simulink model "SIM_PEM"  (R2020b)
settings: Solver=ode23tb  StartTime=0.0  StopTime=3600  RelTol=1e-4  AbsTol=1e-3  EnableMultiTasking=on
undefined symbols (not defined in the file or in its folder): DiscIntNeverNeededParam, FC, FuelCellLoadFcn, gcbh, sps_rtmsupport
libraries: powerlib x16, spsFuelCellModel x1, simulink x1
settings Model: Creator=MathWorks  LastModifiedBy=janluca
settings SolverCC: AutoScaleAbsTol=off
settings DataIOCC: LimitDataPoints=on  SaveFormat=Array  SignalLoggingSaveFormat=ModelDataLogs  ReturnWorkspaceOutputs=off
settings OptimizationCC: ExpressionDepthLimit=2147483647  InitFltsAndDblsToZero=on  EfficientMapNaN2IntZero=off  LifeSpan=inf
settings DebuggingCC: SaveWithParameterizedLinksMsg=none  UnderspecifiedInitializationDetection=Classic  MergeDetectMultiDrivingBlocksExec=none  FcnCallInpInsideContextMsg=warning  AllowSymbolicDim=off  StateNameClashWarn=warning  SFUnexpectedBacktrackingDiag=warning  SFNoUnconditionalDefaultTransitionDiag=warning  SFExecutionAtInitializationDiag=none  ArithmeticOperatorsInVariantConditions=warning
settings HardwareCC: ProdBitPerPointer=32  ProdBitPerSizeT=32  ProdBitPerPtrDiffT=32  ProdLargestAtomicFloat=None  ProdIntDivRoundTo=Undefined  ProdEndianess=Unspecified  ProdWordSize=32  ProdHWDeviceType=32-bit Generic
settings ModelReferenceCC: PropagateSignalLabelsOutOfModel=off
settings SFSimCC: SimUseLocalCustomCode=off  CustomCodeUndefinedFunction=UseInterfaceOnly
settings RTWCC: RTWUseLocalCustomCode=off
settings CodeAppCC: StateflowObjectComments=on
settings GRTTargetCC: TargetFcnLib=ansi_tfl_tmw.mat  TargetLangStandard=C89/C90 (ANSI)  CombineOutputUpdateFcns=off  GRTInterface=on
settings ConfigComp: CovMetricSettings=dw  CovSaveCumulativeToWorkspaceVar=on  CovSaveSingleToWorkspaceVar=on  CovExternalEMLEnable=off  CovSFcnEnable=off
settings SimscapeCC: SimscapeNormalizeSystem=off

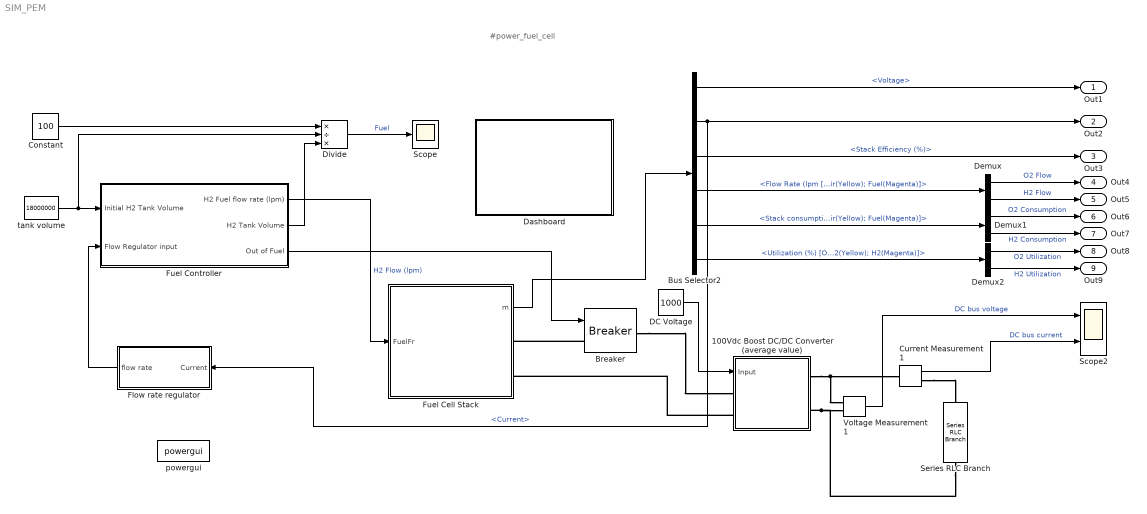
== system SIM_PEM ==
  note: #power_fuel_cell
  100Vdc Boost DC/DC Converter (average value) : Subsystem
  Breaker : powerlib/Elements/Breaker  InitialState=1  SwitchingTimes="[1/60  5/60]"  External=on  BreakerResistance=0.01  SnubberResistance=1e6  SnubberCapacitance=inf  Measurements=None  MoreParameters=on  NoBreakLoop=off
  Bus Selector2 : BusSelector  OutputSignals=Voltage,Current,Stack Efficiency (%),Flow Rate (lpm [Air(Yellow); Fuel(Magenta)],Stack consumption (Standard lpm) [Air(Yellow); Fuel(Magenta)],Utilization (%) [O2(Yellow); H2(Magenta)]
  Constant : Constant  Value=100
  Current Measurement1 : powerlib/Measurements/Current Measurement  PhasorSimulation=off  OutputType=Complex  PSBequivalent=0
  DC Voltage : Constant  Value=1000
  Dashboard : Subsystem
  Demux : Demux  Outputs=2
  Demux1 : Demux  Outputs=2
  Demux2 : Demux  Outputs=2
  Divide : Product  Inputs=*/*
  Flow rate regulator : Subsystem  mask{Nc=96, Uf_H2=99.18, T=65, Pf=1, x=99.95}
      mask prompts: Nc "Number of cells"; Uf_H2 "Nominal Hydrogen utilization (%)"; T "Operating temperature (Celsius)"; Pf "Fuel pressure (bar)"; x "H2 composition (%)"
  Fuel Cell Stack : Subsystem  AncestorBlock=electricdrivelib/Extra Sources/Fuel Cell Stack  DialogController=POWERSYS.PowerSysDialog  LoadFcn=sps_rtmsupport('LoadFcn',gcbh);FuelCellLoadFcn(gcb)  StartFcn=sps_rtmsupport('StartFcn',gcbh);  StopFcn=sps_rtmsupport('StopFcn',gcbh);  mask(Fuel Cell Stack){PresetModel=No (User-Defined), FcType=Proton Exchange Membrane (PEM), Detailed=Detailed, Eoc=[93.2,88], NomVI=[160,65.5], EndVI=[230,58.6], Nc=96, n=54, TOp=65, AirFr=510, SuppPress=[1.26,1], Comp=[99.95,21,1], SignX=off, SignY=off, FlowRateH2=on, FlowRateAir=off, SystemTemp=off, SystemPH2=off, SystemPAir=off, FCDyn=off, FC_tau=0, Peak_O2=80, V_Under=10}
      mask prompts: PresetModel "Preset model:"; FcType "Fuel Cell type:"; Detailed "Model detail Level:"; Eoc "Voltage at 0A and 1A [V_0(V), V_1(V)]"; NomVI "Nominal operating point [Inom(A), Vnom(V)]"; EndVI "Maximum operating point [Iend(A), Vend(V)]"; Nc "Number of cells"; n "Nominal stack efficiency (%)"; TOp "Operating temperature (Celsius)"; AirFr "Nominal Air flow rate (lpm)"; SuppPress "Nominal supply pressure [Fuel (bar), Air (bar)]"; Comp "Nominal composition (%) [H2 O2 H2O(Air)]"; SignX "Fuel  composition [x_H2(%)]"; SignY "Oxidant composition [y_O2(%)]"; FlowRateH2 "Fuel flow rate [FuelFr(lpm)]"; FlowRateAir "Air flow rate [AirFr(lpm)]"; SystemTemp "System Temperature [T(Kelvin)]"; SystemPH2 "Fuel supply pressure [Pfuel(bar)]"; SystemPAir "Air supply pressure [PAir(bar)]"; FCDyn "Specify Fuel Cell Dynamics?"; FC_tau "Fuel Cell response time (sec)"; Peak_O2 "Peak O2 utilization (%)"; V_Under "Voltage undershoot (V) @ peak O2 utilization"
      mask help:
      | Implements a generic hydrogen fuel cell model which allows the simulation for the following types of cells:
      | - Proton Exchange Membrane Fuel Cell (PEMFC)
      | - Solid Oxide Fuel Cell (SOFC)
      | - Alkaline Fuel Cell (AFC)
      mask init:
      | block = gcb;
      | %% DO NOT CHANGE THIS ORDER
      | FuelCellCback(block,'Inputs')
      | [FC, WantBlockChoice, Ts] = FuelCellInit(block,Eoc,NomVI,EndVI,Nc,n,TOp,AirFr,SuppPress,Comp,FlowRateH2,FlowRateAir);
      | powericon('SetInternalModels','set',block,WantBlockChoice);
      settings: CopyFcn=sps_rtmsupport('CopyFcn',gcbh);  DeleteFcn=sps_rtmsupport('DeleteFcn',gcbh);  UndoDeleteFcn=sps_rtmsupport('UndoDeleteFcn',gcbh);  ModelCloseFcn=sps_rtmsupport('ModelCloseFcn',gcbh);  PreSaveFcn=sps_rtmsupport('PreSaveFcn',gcbh);  PostSaveFcn=sps_rtmsupport('PostSaveFcn',gcbh);  NameChangeFcn=sps_rtmsupport('NameChangeFcn',gcbh);  PreCopyFcn=sps_rtmsupport('PreCopyFcn',gcbh);  OpenFcn=sps_rtmsupport('OpenFcn',gcbh, [1 2 3 13 14 15 16 17 18 19 20]);  CloseFcn=sps_rtmsupport('CloseFcn',gcbh);  PreDeleteFcn=sps_rtmsupport('PreDeleteFcn',gcbh);
      mask Help: helpview(psbhelp)
      mask TypeOptions PresetModel: No (User-Defined) | PEMFC - 1.26 kW - 24 Vdc | PEMFC - 6 kW - 45 Vdc | PEMFC - 50 kW - 625 Vdc | AFC - 2.4 kW - 48 Vdc | SOFC - 3 kW - 100 Vdc | SOFC - 25 kW - 630 Vdc
      mask Callback PresetModel: FuelCellCback(gcb,'Preset')
      mask TypeOptions Detailed: Simplified | Detailed
      mask Callback Detailed: FuelCellCback(gcb,'Visibilities')
      mask Callback FlowRateAir: FuelCellCback(gcb,'Visibilities')
      mask Callback FCDyn: FuelCellCback(gcb,'Visibilities')
      mask DialogControl ParameterTabVar0 Prompt: Parameters
      mask DialogControl plot_graph Prompt: Plot V_I characteristic
      mask DialogControl plot_graph Callback: FuelCellCback(gcb,'PlotGraph');
      mask DialogControl ViewParam Prompt: View Cell parameters
      mask DialogControl ViewParam Callback: FuelCellCback(gcb,'ViewParam');
      mask DialogControl ParameterTabVar01 Prompt: Signal variation
      mask DialogControl ParameterTabVar012 Prompt: Fuel Cell Dynamics
      mask Display: image(imread('power_fuelcell.png'));
  Fuel Controller : Subsystem
  Scope : Scope
  Scope2 : Scope  NumInputPorts=2
  Series RLC Branch : powerlib/Elements/Series RLC Branch  LConnTagsString=__new0  RConnTagsString=__new0  BranchType=R  Resistance=150  Inductance=100*100/6000  SetiL0=off  InitialCurrent=0  Capacitance=1e-6  Setx0=off  InitialVoltage=0  Measurements=None
  Voltage Measurement1 : powerlib/Measurements/Voltage Measurement  PhasorSimulation=off  OutputType=Complex  PSBequivalent=0
  powergui : powerlib/powergui  SimulationMode=Continuous  SampleTime=1e-5  frequency=50  Iterations=50  frequencyindice=0  Pbase=100e6  ErrMax=1e-4  UnitsV=kV  UnitsW=MW  buscounter=0  FunctionMessages=off  echomessages=off  EnableUseOfTLC=off  CurrentSourceSwitches=off  DisableSnubberDevices=off  DisableRonSwitches=off  DisableVfSwitches=off  DisplayEquations=off  AutomaticDiscreteSolvers=off  SolverType=Tustin  Interpol=off  ExternalGateDelay=off  methode=off  Ts=0  x0status=blocks  SPID=off  SwTol=0  HookPort=off  NonlinearTolerance=1e-4  nMaxIteration=100  ContinueOnMaxIteration=off  RestoreLinks=warning  ResistiveCurrentMeasurement=off  Frange=[0:2:500]  Ylog=off  Xlog=on  ShowGrid=off  save=off  variable=ZData  structure=0  ZoomFFT=on  StartTime=0.0  cycles=1  DisplayStyle=1  fundamental=60  FreqAxis=off  MaxFrequency=1000  frequencyindicesteady=1  RmsSteady=1  display=off
  tank volume : Constant  Value=18000000
  Out1 : Outport  SignalName=Stack Voltage
  Out2 : Outport  Port=2  SignalName=Stack Current
  Out3 : Outport  Port=3  SignalName=Stack Efficiency
  Out4 : Outport  Port=4  SignalName=O2 Flow
  Out5 : Outport  Port=5  SignalName=H2 Flow
  Out6 : Outport  Port=6  SignalName=O2 Consumption
  Out7 : Outport  Port=7  SignalName=H2 Consumption
  Out8 : Outport  Port=8  SignalName=O2 Utilization
  Out9 : Outport  Port=9  SignalName=H2 Utilization
  wires:
  Fuel Cell Stack/1(m) -> Bus Selector2/1
  Current Measurement1/1 -> Scope2/2  "DC bus current"
  Fuel Controller/1(H2 Fuel flow rate (lpm)) -> Fuel Cell Stack/1(FuelFr)  "H2 Flow (lpm)"
  tank volume/1 -> Divide/2, Fuel Controller/1(Initial H2 Tank Volume)
  Flow rate regulator/1(flow rate) -> Fuel Controller/2(Flow Regulator input)
  Fuel Controller/3(Out of Fuel) -> Breaker/1
  Bus Selector2/4 -> Demux/1  "<Flow Rate (lpm [Air(Yellow); Fuel(Magenta)]>"
  Bus Selector2/5 -> Demux1/1  "<Stack consumption (Standard lpm) [Air(Yellow); Fuel(Magenta)]>"
  Bus Selector2/6 -> Demux2/1  "<Utilization (%) [O2(Yellow); H2(Magenta)]>"
  Bus Selector2/1 -> Out1/1  "<Voltage>"
  Bus Selector2/2 -> Out2/1, Flow rate regulator/1(Current)  "<Current>"
  Bus Selector2/3 -> Out3/1  "<Stack Efficiency (%)>"
  Demux/1 -> Out4/1  "O2 Flow"
  Demux/2 -> Out5/1  "H2 Flow"
  Demux1/1 -> Out6/1  "O2 Consumption"
  Demux1/2 -> Out7/1  "H2 Consumption"
  Demux2/1 -> Out8/1  "O2 Utilization"
  Demux2/2 -> Out9/1  "H2 Utilization"
  Divide/1 -> Scope/1  "Fuel"
  Fuel Controller/2(H2 Tank Volume) -> Divide/3
  Constant/1 -> Divide/1
  Voltage Measurement1/1 -> Scope2/1  "DC bus voltage"
  DC Voltage/1 -> 100Vdc Boost DC/DC Converter (average value)/1(Input)
  connections:
  100Vdc Boost DC/DC Converter (average value)/RConn2 -- Series RLC Branch/RConn1 -- Voltage Measurement1/LConn2
  Current Measurement1/RConn1 -- Series RLC Branch/LConn1
  100Vdc Boost DC/DC Converter (average value)/LConn2 -- Fuel Cell Stack/RConn2
  Breaker/RConn1 -- 100Vdc Boost DC/DC Converter (average value)/LConn1
  100Vdc Boost DC/DC Converter (average value)/RConn1 -- Current Measurement1/LConn1 -- Voltage Measurement1/LConn1
  Breaker/LConn1 -- Fuel Cell Stack/RConn1

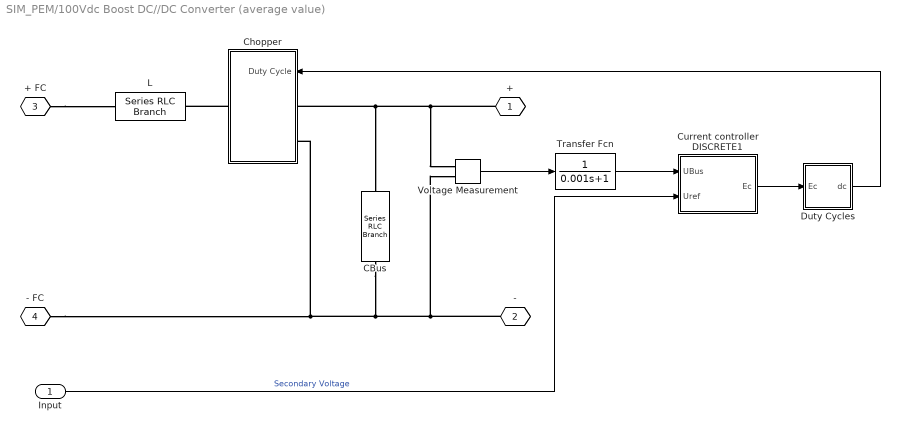
== system SIM_PEM/100Vdc Boost DC//DC Converter (average value) ==
  Input : Inport
  CBus : powerlib/Elements/Series RLC Branch  LConnTagsString=__new0  RConnTagsString=__new0  BranchType=RC  Resistance=0.2  Inductance=1e-3  SetiL0=off  InitialCurrent=0  Capacitance=7500e-6  Setx0=on  InitialVoltage=100  Measurements=None
  Chopper : Subsystem  mask(SPSdrives Converter){SnubberResistance=10e3, SnubberCapacitance=inf, Ron=1e-3, ForwardVoltages=[1.3,1.3], IGBTParameters=[0,0], converterType=Inverter}
      mask prompts: SnubberResistance "Snubber resistance Rs (Ohms):"; SnubberCapacitance "Snubber capacitance Cs (F):"; Ron "Ron (Ohms):"; ForwardVoltages "Forward voltages [Device Vf(V), Diode Vd (V)]"; IGBTParameters "[Tf(s), Tt(s)]:"; converterType "Converter type:"
      mask help: This model implements an average-value buck converter."Duty Cycle" contains the duty cycle of the internal IGBT device.
      mask TypeOptions converterType: Rectifier | Inverter
      mask Display: plot(0,0,100,100,[39 39 23.8],[71 28 28],[44 56 49.6 56 52.8 56 61 61],[39.2 33.6 32.8 33.6 40.8 33.6 30 12.4],[44 44 44 61 61],[28 71 60 66.4 90],[75 67 83 75 67 83 75 75],[54 42 42 54 54 54 54 66],[61 75 75],[24 24 42],[75 75 61],[66,76,76])
  Current controller DISCRETE1 : Subsystem  mask(PI controller){Kp=0.0005, Ki=0.15, Ts=1e-3}
      mask prompts: Kp "Proportional gain (Kp)"; Ki "Integral gain (Ki)"; Ts "Sample time (s) :"
      mask help: Proportional-Integral Speed Controller
      mask Display: plot(0,0,100,100,[35,35,65],[70,30,30],[35,65],[45,60])
  Duty Cycles : Subsystem
  L : powerlib/Elements/Series RLC Branch  LConnTagsString=__new0  RConnTagsString=__new0  BranchType=L  Resistance=0.3  Inductance=500e-6  SetiL0=off  InitialCurrent=0  Capacitance=100e-6  Setx0=off  InitialVoltage=0  Measurements=None
  Transfer Fcn : TransferFcn  Denominator=[0.001 1]
  Voltage Measurement : powerlib/Measurements/Voltage Measurement  PhasorSimulation=off  OutputType=Complex  PSBequivalent=0
  + : PMIOPort  Tag=PMCPort  Side=Right
  - : PMIOPort  Tag=PMCPort  Port=2  Side=Right
  + FC : PMIOPort  Tag=PMCPort  Port=3  Side=Left
  - FC : PMIOPort  Tag=PMCPort  Port=4  Side=Left
  wires:
  Input/1 -> Current controller DISCRETE1/2(Uref)  "Secondary Voltage"
  Voltage Measurement/1 -> Transfer Fcn/1
  Duty Cycles/1(dc) -> Chopper/1(Duty Cycle)
  Transfer Fcn/1 -> Current controller DISCRETE1/1(UBus)
  Current controller DISCRETE1/1(Ec) -> Duty Cycles/1(Ec)
  connections:
  - FC/RConn1 -- Voltage Measurement/LConn2 -- -/RConn1 -- CBus/RConn1 -- Chopper/LConn2
  Voltage Measurement/LConn1 -- +/RConn1 -- Chopper/LConn1 -- CBus/LConn1
  Chopper/RConn1 -- L/LConn1
  + FC/RConn1 -- L/RConn1

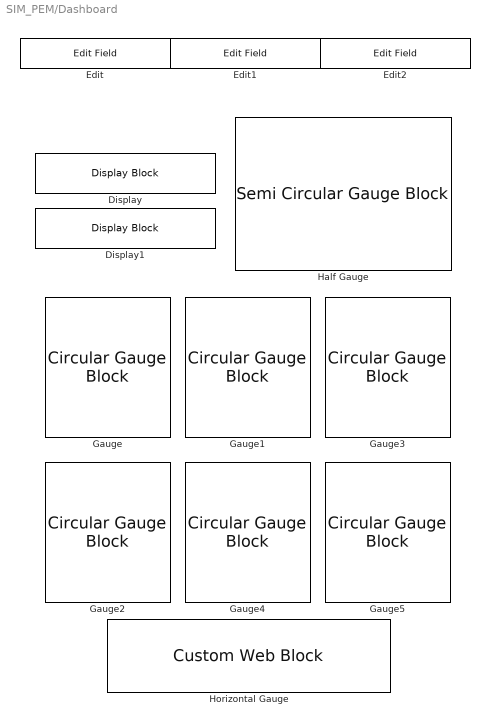
== system SIM_PEM/Dashboard ==
  Display : DisplayBlock  LabelPosition=Hide  Format=Custom  Transparency=1  FormatString=%.2f V
  Display1 : DisplayBlock  LabelPosition=Hide  Format=Custom  Transparency=1  FormatString=%.2f A
  Edit : EditField  LabelPosition=Hide  ShowInitialText=on  Alignment=Center
  Edit1 : EditField  LabelPosition=Hide  ShowInitialText=on  Alignment=Center
  Edit2 : EditField  LabelPosition=Hide  ShowInitialText=on  Alignment=Center
  Gauge : CircularGaugeBlock  ScaleMax=750
  Gauge1 : CircularGaugeBlock  ScaleMax=500
  Gauge2 : CircularGaugeBlock  ScaleMax=250
  Gauge3 : CircularGaugeBlock
  Gauge4 : CircularGaugeBlock  ScaleMax=250
  Gauge5 : CircularGaugeBlock
  Half Gauge : SemiCircularGaugeBlock  ScaleMax=60
  Horizontal Gauge : CustomWebBlock  ShowInitialText=on  Configuration="{\"components\":[{\"name\":\"LinearScaleComponent\",\"settings\":{\"bounds\":{\"max\":100,\"min\":0,\"tickInterval\":\"auto\"},\"internalTickHeightScaleFactor\":0.5,\"labelColor\":[250,245,199],\"labelFont\":{\"font\":\"Arial\",\"fontSize\":12},\"labelTransparency\":1,\"needleImage\":{\"size\":[21,75],\"src\":\"data:image\\/svg+xml;base64,PHN2ZyB4bWxucz0iaHR0cDovL3d3dy53My5vcmcvMjAwMC9zdmciIHhtbG5zOnhsaW5rPSJodHRwOi8vd3d3LnczLm9yZy8xOTk5L3hsaW5rIiB2aWV3Qm94PSIwIDAgMjEgNzUiPjxkZWZzPjxzdHlsZT4uY2xzLTF7ZmlsbDpub25lO30uY2xzLTJ7aXNvbGF0aW9uOmlzb2xhdGU7fS5jbHMtM3tjbGlwLXBhdGg6dXJsKCNjbGlwLXBhdGgpO30uY2xzLTR7b3BhY2l0eTowLjM7bWl4LWJsZW5kLW1vZGU6bXVsdGlwbHk7fS5jbHMtNXtmaWxsOiNlYjI2Mjk7fTwvc3R5bGU+PGNsaXBQYXRoIGlkPSJjbGlwLXBhdGgiIHRyYW5zZm9y ...(+1928 chars)\",\"srcOrientation\":\"horizontal\"},\"needleOffset\":[0,0.01094391244870041],\"needleSize\":{\"height\":0.7589285714285714,\"width\":0.11960078534031414},\"position\":[0.06986607142857143,0.01995798319327731,0.9641544117647058,0.8],\"scaleColors\":[],\"scaleColorsSize\":0.2,\"showLabels\":1,\"showMinorTicks\":0,\"showSpanLine\":1,\"showTicks\":1,\"tickColor\":[250,245,200],\"tickTransparency\":1,\"valueBarColor\":[23,89,176],\"valueBarOffset\":0,\"valueBarSize\":0.23,\"valueBarTransparency\":1}},{\"name\":\"BackgroundImageComponent\",\"settings\":{\"image\":{\"size\":[380,101],\"src\":\"data:image\\/svg+xml;base64,PHN2ZyB4bWxucz0iaHR0cDovL3d3dy53My5vcmcvMjAwMC9zdmciIHZpZXdCb3g9IjAgMCAzODAgMTAxIj48ZGVmcz48c3R5bGU+LmNscy0xe2ZpbGw6IzAwMmI0Mjt9LmNscy0ye2ZpbGw6IzQyNzA4Mjt9LmNscy0ze2ZpbGw6IzdjYTBiMjt9PC9zdHlsZT48L2RlZnM+PHRpdGxlPmhvcml6b250YWxfZ2F1Z2VfIGJhY2tncm91bmQ8L3RpdGxlPjxnIGlkPSJMYXllcl8yIiBkYXRhLW5hbWU9IkxheWVyIDIiPjxnIGlkPSJMYXllcl8xLTIiIGRhdGEtbmFtZT0iTGF5ZXIgMSI+PHJlY3QgY2xhc3M9ImNscy0xIiB4PSIxMSIgeT0iMTEiIHdpZHRoPSIzNTgiIGhlaWdodD0iNzkiLz48cGF0aCBjbGFzcz0iY2xzLTIiIGQ9Ik04LDhWOTNIMzcyVjhaTTM2OSw5MEgxMVYxMUgzNjlaIi8+PHBhdGggY2xhc3M9ImNscy0zIiBkPSJNMCwwVjEwMUgzODBWMFpNMzcyLDkzSDhWOEgzNzJaIi8+PC9nPjwvZz48L3N2Zz4=\",\"srcOrientation\":\"horizontal\"},\"position\":[0,0,1,1],\"scaleMode\":\"0\"}},{\"name\":\"ForegroundImageComponent\",\"settings\":{\"image\":{\"size\":[0,0],\"src\":\"default\",\"srcOrientation\":[]},\"isForeground\":1,\"position\":[0,0,1,1],\"scaleMode\":\"0\"}}],\"settings\":{\"BindingType\":\"signal\",\"aspectRatio\":3.7777777777777777,\"fixedAspectRatio\":\"on\",\"orientation\":\"horizontal\"},\"type\":\"LinearGauge\"}"

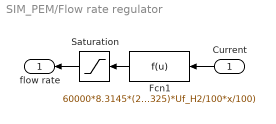
== system SIM_PEM/Flow rate regulator ==
  Current : Inport
  Fcn1 : Fcn  Expr=60000*8.3145*(273+T)*Nc*u(1)/(2*96485*(Pf*101325)*Uf_H2/100*x/100)
  Saturation : Saturate  UpperLimit=inf  LowerLimit=1
  flow rate : Outport  VectorParamsAs1DForOutWhenUnconnected=off
  wires:
  Fcn1/1 -> Saturation/1
  Current/1 -> Fcn1/1
  Saturation/1 -> flow rate/1

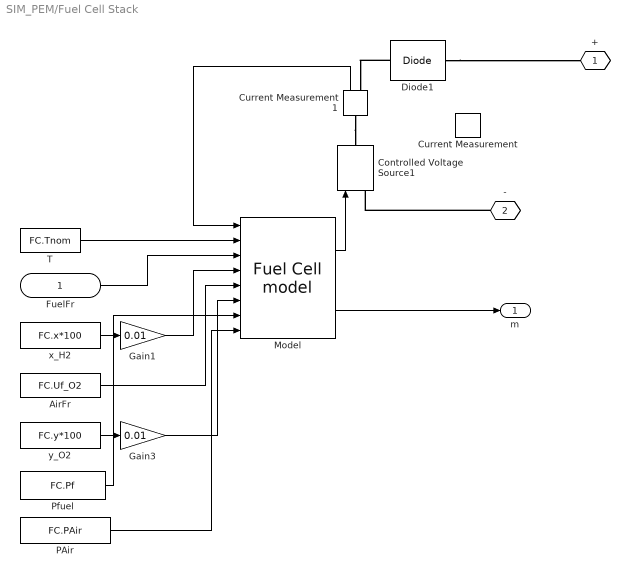
== system SIM_PEM/Fuel Cell Stack ==
  FuelFr : Inport
  AirFr : Constant  Value=FC.Uf_O2
  Controlled Voltage Source1 : powerlib/Electrical Sources/Controlled Voltage Source  Initialize=on  Source_Type=AC  Amplitude=0  Phase=0  Frequency=0  Measurements=None
  Current Measurement : powerlib/Measurements/Current Measurement  PhasorSimulation=off  OutputType=Complex  PSBequivalent=0
  Current Measurement1 : powerlib/Measurements/Current Measurement  PhasorSimulation=off  OutputType=Complex  PSBequivalent=0
  Diode1 : powerlib/Power Electronics/Diode  Ron=FC.Rohm  Lon=0  Vf=0  IC=0  UseSnubber=off  Rs=1e4  Cs=inf  Measurements=off
  Gain1 : Gain  Gain=0.01
  Gain3 : Gain  Gain=0.01
  Model : spsFuelCellModel/Fuel Cell model  SystemSampleTime=-1  LabelModeActiveChoice=Continuous/Detailed  VariantActivationTime=update diagram  Latency=0  AutoFrameSizeCalculation=off
      settings: AttributesFormatString=%<BlockChoice>  SourceProductBaseCode=PS
  PAir : Constant  Value=FC.PAir
  Pfuel : Constant  Value=FC.Pf
  T : Constant  Value=FC.Tnom
  x_H2 : Constant  Value=FC.x*100
  y_O2 : Constant  Value=FC.y*100
  + : PMIOPort  Tag=PMCPort  Side=Right
  - : PMIOPort  Tag=PMCPort  Port=2  Side=Right
  m : Outport  VectorParamsAs1DForOutWhenUnconnected=off
  wires:
  PAir/1 -> Model/8
  Pfuel/1 -> Model/7
  T/1 -> Model/2
  Model/1 -> Controlled Voltage Source1/1
  Current Measurement1/1 -> Model/1
  Model/2 -> m/1
  FuelFr/1 -> Model/3
  x_H2/1 -> Gain1/1
  AirFr/1 -> Model/5
  y_O2/1 -> Gain3/1
  Gain1/1 -> Model/4
  Gain3/1 -> Model/6
  connections:
  Current Measurement1/LConn1 -- Controlled Voltage Source1/RConn1
  Diode1/LConn1 -- Current Measurement1/RConn1
  -/RConn1 -- Controlled Voltage Source1/LConn1
  Diode1/RConn1 -- +/RConn1

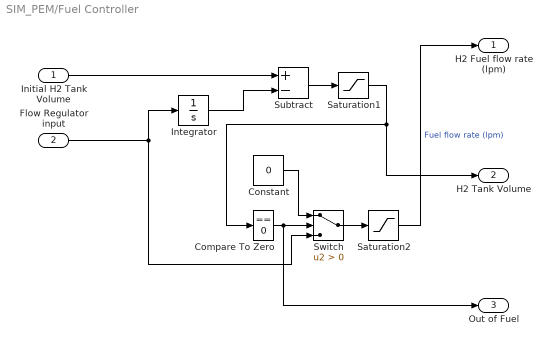
== system SIM_PEM/Fuel Controller ==
  Initial H2 Tank Volume : Inport
  Flow Regulator input : Inport  Port=2
  Compare To Zero : simulink/Logic and Bit Operations/Compare To Zero  relop===  OutDataTypeStr=boolean
  Constant : Constant  Value=0
  Integrator : Integrator
  Saturation1 : Saturate  UpperLimit=inf  LowerLimit=0
  Saturation2 : Saturate  UpperLimit=154  LowerLimit=0
  Subtract : Sum  Inputs=+-
  Switch : Switch  Criteria=u2 > Threshold
  H2 Fuel flow rate (lpm) : Outport
  H2 Tank Volume : Outport  Port=2
  Out of Fuel : Outport  Port=3
  wires:
  Constant/1 -> Switch/1
  Initial H2 Tank Volume/1 -> Subtract/1
  Switch/1 -> Saturation2/1
  Compare To Zero/1 -> Switch/2, Out of Fuel/1
  Saturation1/1 -> H2 Tank Volume/1, Compare To Zero/1
  Saturation2/1 -> H2 Fuel flow rate (lpm)/1  "Fuel flow rate (lpm)"
  Subtract/1 -> Saturation1/1
  Integrator/1 -> Subtract/2
  Flow Regulator input/1 -> Switch/3, Integrator/1

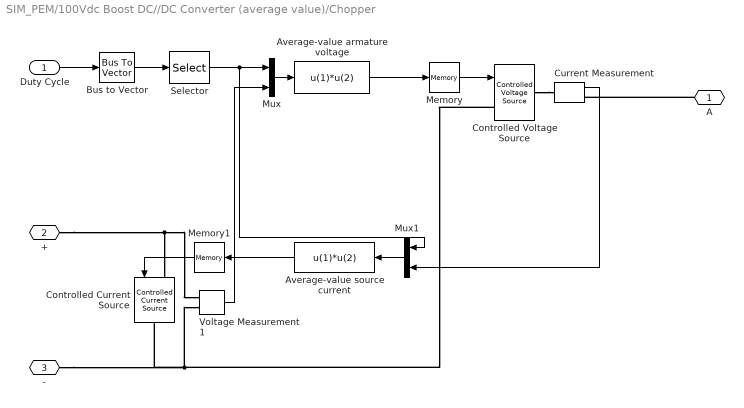
== system SIM_PEM/100Vdc Boost DC//DC Converter (average value)/Chopper ==
  Duty Cycle : Inport
  Average-value armature voltage : Fcn  Expr=u(1)*u(2)
  Average-value source current : Fcn  Expr=u(1)*u(2)
  Bus to Vector : BusToVector
  Controlled Current Source : powerlib/Electrical Sources/Controlled Current Source  Initialize=on  Source_Type=AC  Amplitude=0  Phase=0  Frequency=0  Measurements=None
  Controlled Voltage Source : powerlib/Electrical Sources/Controlled Voltage Source  Initialize=on  Source_Type=AC  Amplitude=0  Phase=0  Frequency=0  Measurements=None
  Current Measurement : powerlib/Measurements/Current Measurement  Tag=PoWeRsYsTeMmEaSuReMeNt  PhasorSimulation=off  OutputType=Magnitude  PSBequivalent=0
  Memory : Memory
  Memory1 : Memory
  Mux : Mux  Inputs=2
  Mux1 : Mux  Inputs=2
  Selector : Selector  InputPortWidth=2  IndexOptions=Index vector (dialog)  Indices=[1]  OutputSizes=1
  Voltage Measurement1 : powerlib/Measurements/Voltage Measurement  Tag=PoWeRsYsTeMmEaSuReMeNt  PhasorSimulation=off  OutputType=Magnitude  PSBequivalent=0
  A : PMIOPort  Side=Right
  + : PMIOPort  Port=2  Side=Left
  - : PMIOPort  Port=3  Side=Left
  wires:
  Selector/1 -> Mux1/1, Mux/1
  Memory1/1 -> Controlled Current Source/1
  Average-value source current/1 -> Memory1/1
  Current Measurement/1 -> Mux1/2
  Mux1/1 -> Average-value source current/1
  Duty Cycle/1 -> Bus to Vector/1
  Voltage Measurement1/1 -> Mux/2
  Mux/1 -> Average-value armature voltage/1
  Average-value armature voltage/1 -> Memory/1
  Memory/1 -> Controlled Voltage Source/1
  Bus to Vector/1 -> Selector/1
  connections:
  A/RConn1 -- Current Measurement/RConn1
  Controlled Voltage Source/RConn1 -- Current Measurement/LConn1
  +/RConn1 -- Voltage Measurement1/LConn1 -- Controlled Current Source/LConn1
  Controlled Voltage Source/LConn1 -- -/RConn1 -- Controlled Current Source/RConn1 -- Voltage Measurement1/LConn2

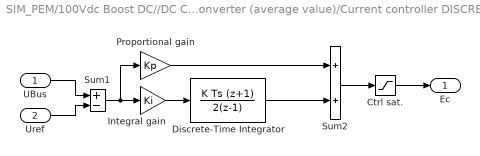
== system SIM_PEM/100Vdc Boost DC//DC Converter (average value)/Current controller DISCRETE1 ==
  UBus : Inport
  Uref : Inport  Port=2
  Ctrl sat. : Saturate  UpperLimit=0.95  LowerLimit=-0.95
  Discrete-Time Integrator : DiscreteIntegrator  IntegratorMethod=Integration: Trapezoidal  SampleTime=Ts  LimitOutput=on  UpperSaturationLimit=0.95  LowerSaturationLimit=-0.95  ICPrevOutput=DiscIntNeverNeededParam  ICPrevScaledInput=DiscIntNeverNeededParam
  Integral gain : Gain  Gain=Ki  SaturateOnIntegerOverflow=on  OutDataTypeStr=Inherit: Same as input  ParamDataTypeStr=Inherit: Same as input
  Proportional gain : Gain  Gain=Kp  SaturateOnIntegerOverflow=on  OutDataTypeStr=Inherit: Same as input  ParamDataTypeStr=Inherit: Same as input
  Sum1 : Sum  Inputs=+-  InputSameDT=on  SaturateOnIntegerOverflow=on  OutDataTypeStr=Inherit: Same as first input
  Sum2 : Sum  InputSameDT=on  SaturateOnIntegerOverflow=on  OutDataTypeStr=Inherit: Same as first input
  Ec : Outport  InitialOutput=0  VectorParamsAs1DForOutWhenUnconnected=off
  wires:
  Ctrl sat./1 -> Ec/1
  Sum2/1 -> Ctrl sat./1
  Discrete-Time Integrator/1 -> Sum2/2
  Uref/1 -> Sum1/2
  UBus/1 -> Sum1/1
  Sum1/1 -> Proportional gain/1, Integral gain/1
  Integral gain/1 -> Discrete-Time Integrator/1
  Proportional gain/1 -> Sum2/1

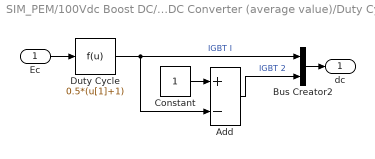
== system SIM_PEM/100Vdc Boost DC//DC Converter (average value)/Duty Cycles ==
  Ec : Inport
  Add : Sum  Inputs=+-
  Bus Creator2 : BusCreator  Inputs=2
  Constant : Constant
  Duty Cycle : Fcn  Expr=0.5*(u[1]+1)
  dc : Outport  VectorParamsAs1DForOutWhenUnconnected=off
  wires:
  Bus Creator2/1 -> dc/1
  Ec/1 -> Duty Cycle/1
  Constant/1 -> Add/1
  Add/1 -> Bus Creator2/2  "IGBT 2"
  Duty Cycle/1 -> Bus Creator2/1, Add/2  "IGBT I"
